simulink model "simulation_pdx_v2"  (R2015a)
settings: Solver=ode45  StartTime=0.0  StopTime=2000.0  RelTol=1e-3
values from neighbouring files (symbols this model uses):
  g = 1.6    [InitialParameters.m]
  M0 = 15000 - MFuel0    (= 7000)    [InitialParameters.m]
libraries: simulink x1
settings Model: Creator=MateusVendramini  LastModifiedBy=MateusVendramini
settings SolverCC: AlgebraicLoopSolver=LineSearch

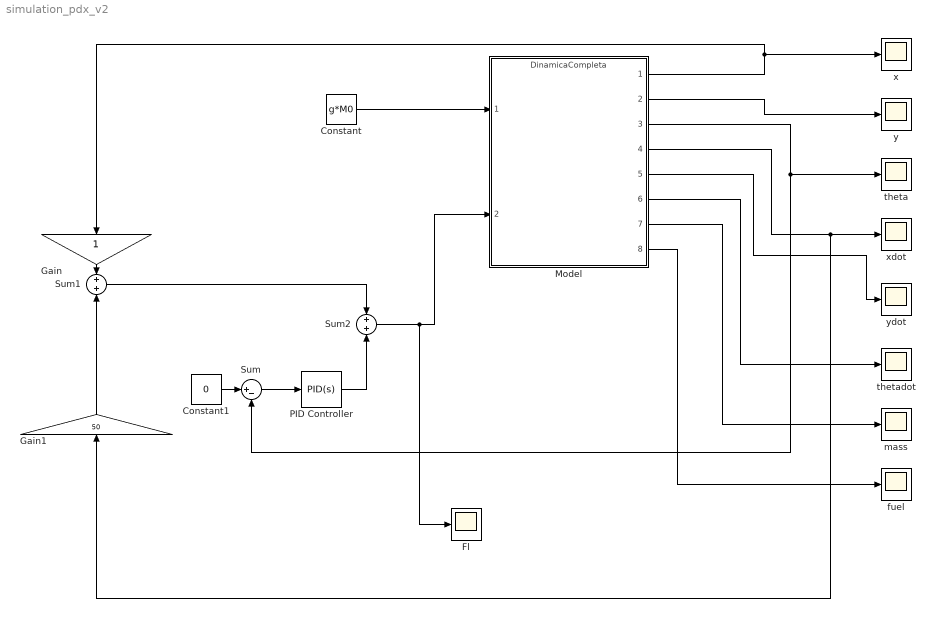
== system simulation_pdx_v2 ==
  Constant : Constant  Value=g*M0
  Constant1 : Constant  Value=0
  Fl : Scope
      settings: SaveName=ScopeData8
  Gain : Gain
  Gain1 : Gain  Gain=50
  Model : ModelReference  ModelNameDialog=DinamicaCompleta.slx  SimulationMode=Normal  ModelReferenceVersion=1.4  CopyOfModelName=DinamicaCompleta.slx  DefaultDataLogging=on
  PID Controller : simulink/Continuous/PID Controller  Controller=PID  TimeDomain=Continuous-time  SampleTime=-1  IntegratorMethod=Forward Euler  FilterMethod=Forward Euler  Form=Parallel  UseFilter=on  ControllerParametersSource=internal  P=2003  I=0  D=8510  N=50  InitialConditionSource=internal  InitialConditionForIntegrator=0  InitialConditionForFilter=0  ExternalReset=none  LimitOutput=off  UpperSaturationLimit=inf  LowerSaturationLimit=-inf  LinearizeAsGain=on  AntiWindupMode=none  Kb=1  TrackingMode=off  Kt=1  PParamMin=[]  PParamMax=[]  IParamMin=[]  IParamMax=[]  DParamMin=[]  DParamMax=[]  NParamMin=[]  NParamMax=[]  KbParamMin=[]  KbParamMax=[]  KtParamMin=[]  KtParamMax=[]  POutMin=[]  POutMax=[]  IOutMin=[]  IOutMax=[]  DOutMin=[]  DOutMax=[]  NOutMin=[]  NOutMax=[]  KbOutMin=[]  KbOutMax=[]  KtOutMin=[]  KtOutMax=[]  IntegratorOutMin=[]  IntegratorOutMax=[]  FilterOutMin=[]  FilterOutMax=[]  SumOutMin=[]  SumOutMax=[]  SumI1OutMin=[]  SumI1OutMax=[]  SumI2OutMin=[]  SumI2OutMax=[]  SumI3OutMin=[]  SumI3OutMax=[]  SumDOutMin=[]  SumDOutMax=[]  SaturationOutMin=[]  SaturationOutMax=[]  IntegratorContinuousStateAttributes=''  IntegratorStateMustResolveToSignalObject=off  IntegratorRTWStateStorageClass=Auto  FilterContinuousStateAttributes=''  FilterStateMustResolveToSignalObject=off  FilterRTWStateStorageClass=Auto  DifferentiatorICPrevScaledInput=0  DifferentiatorOutMin=[]  DifferentiatorOutMax=[]
  Sum : Sum  Inputs=|+-
  Sum1 : Sum  Inputs=+|+
  Sum2 : Sum  Inputs=+|+
  fuel : Scope
      settings: SaveName=ScopeData7
  mass : Scope
      settings: SaveName=ScopeData6
  theta : Scope
      settings: SaveName=ScopeData2
  thetadot : Scope
      settings: SaveName=ScopeData5
  x : Scope
      settings: YMin=-100  YMax=90
  xdot : Scope
      settings: SaveName=ScopeData3
  y : Scope
  ydot : Scope
      settings: SaveName=ScopeData4
  wires:
  Sum/1 -> PID Controller/1
  Constant/1 -> Model/1
  Model/3 -> theta/1, Sum/2
  Model/1 -> x/1, Gain/1
  Model/2 -> y/1
  Model/4 -> xdot/1, Gain1/1
  Model/5 -> ydot/1
  Model/6 -> thetadot/1
  Model/7 -> mass/1
  Model/8 -> fuel/1
  Gain1/1 -> Sum1/2
  Gain/1 -> Sum1/1
  Sum1/1 -> Sum2/1
  PID Controller/1 -> Sum2/2
  Sum2/1 -> Fl/1, Model/2
  Constant1/1 -> Sum/1
